simulink model "c2000_encode_decode_packet"  (R2021b)
settings: Solver=FixedStepDiscrete  StartTime=0.0  StopTime=Inf  RelTol=1e-3  EnableMultiTasking=on
undefined symbols (not defined in the file or in its folder): CR
libraries: embeddedblockslib x2, c280xlib x2, demo_controls x1
settings Model: ExtModeTrigDuration=8  Creator=The MathWorks, Inc.  LastModifiedBy=The MathWorks, Inc.
settings DataIOCC: ReturnWorkspaceOutputs=off
settings OptimizationCC: DefaultUnderspecifiedDataType=single  EnhancedBackFolding=on  PassReuseOutputArgsAs=Individual arguments  MaxStackSize=1024  OptimizeBlockOrder=speed  DifferentSizesBufferReuse=on  OptimizationCustomize=off  DenormalBehavior=FlushToZero  EfficientTunableParamExpr=on
settings DebuggingCC: ParameterPrecisionLossMsg=none  ParameterTunabilityLossMsg=error
settings HardwareCC: ProdBitPerChar=16  ProdBitPerInt=16  ProdBitPerPointer=32  ProdBitPerSizeT=32  ProdBitPerPtrDiffT=32  ProdLargestAtomicInteger=Integer  ProdLargestAtomicFloat=None  ProdWordSize=16  ProdLongLongMode=on  ProdHWDeviceType=Texas Instruments->C2000
settings ModelReferenceCC: ModelReferenceNumInstancesAllowed=Single
settings SFSimCC: MATLABDynamicMemAlloc=off
settings RTWCC: Description=Embedded Coder  SystemTargetFile=ert.tlc  HardwareBoard=TI Delfino F28379D LaunchPad  TemplateMakefile=ert_default_tmf  Toolchain=Texas Instruments Code Composer Studio (C2000)  BuildConfiguration=Faster Runs
settings CodeAppCC: ForceParamTrailComments=on  IgnoreCustomStorageClasses=off  OperatorAnnotations=on  SimulinkDataObjDesc=on  SFDataObjDesc=on  InsertBlockDesc=on
settings ERTTargetCC: CodeReplacementLibrary=TI C28x  ExtModeTransport=4  ExtModeStaticAlloc=on  ExtModeStaticAllocSize=10000  ExtModeMexFile=ext_xcp  ExtModeIntrfLevel=Level2 - Open

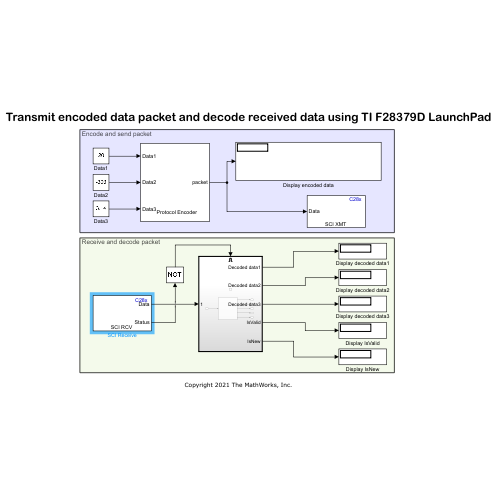
[thumbnail: Simulink's stored preview of the top-level diagram]
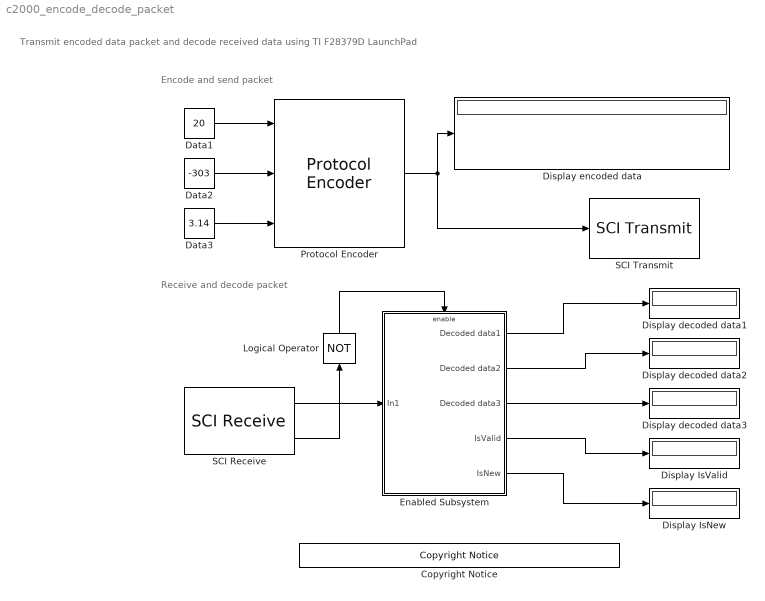
== system c2000_encode_decode_packet ==
  note: Receive and decode packet
  note: Transmit encoded data packet and decode received data using TI F28379D LaunchPad
  note: Encode and send packet
  Copyright Notice : demo_controls/Copyright Notice  year=2021  prod=tic6000
      settings: SourceProductBaseCode=ME
  Data1 : Constant  Value=20  OutDataTypeStr=uint8
  Data2 : Constant  Value=-303  OutDataTypeStr=int16
  Data3 : Constant  Value=3.14  OutDataTypeStr=single  LockScale=on
  Display IsNew : Display
  Display IsValid : Display
  Display decoded data1 : Display
  Display decoded data2 : Display
  Display decoded data3 : Display
  Display encoded data : Display
  Enabled Subsystem : Subsystem  TreatAsAtomicUnit=on
  Logical Operator : Logic  Operator=NOT  AllPortsSameDT=off  OutDataTypeStr=boolean
  Protocol Encoder : embeddedblockslib/Protocol Encoder  Header=36  FieldTable={ 'Data1', '1', 'uint8', 'Little endian'; 'Data2', '1', 'int16', 'Little endian'; 'Data3', '1', 'single', 'Little endian' }  IsChecksumRequired=on  ChecksumAlgorithm=XOR of bytes  ChecksumSize=[]  TerminatorOption=CR ('\r')  CustomTerminatorVal=[]
      settings: SourceProductBaseCode=ARDUINO,TIC2000
  SCI Receive : c280xlib/SCI Receive  sciModule=B  dataHead=''  dataTail=''  dataType=uint8  dataDim=10  initValue=0  errOption=Output the last received value  errValue=0  sampleTime=0.1  outputStatus=on  postInterrupt=off  numFifo=1
      settings: SourceProductBaseCode=TIC2000
  SCI Transmit : c280xlib/SCI Transmit  sciModule=B  dataHead=''  dataTail=''  postInterrupt=off  numFifo=1
  wires:
  Enabled Subsystem/3(Decoded data3) -> Display decoded data3/1
  Enabled Subsystem/1(Decoded data1) -> Display decoded data1/1
  Protocol Encoder/1 -> SCI Transmit/1, Display encoded data/1
  Enabled Subsystem/5(IsNew) -> Display IsNew/1
  Data3/1 -> Protocol Encoder/3
  Data1/1 -> Protocol Encoder/1
  Enabled Subsystem/4(IsValid) -> Display IsValid/1
  Enabled Subsystem/2(Decoded data2) -> Display decoded data2/1
  Data2/1 -> Protocol Encoder/2
  Logical Operator/1 -> Enabled Subsystem/Enable
  SCI Receive/1 -> Enabled Subsystem/1(In1)
  SCI Receive/2 -> Logical Operator/1

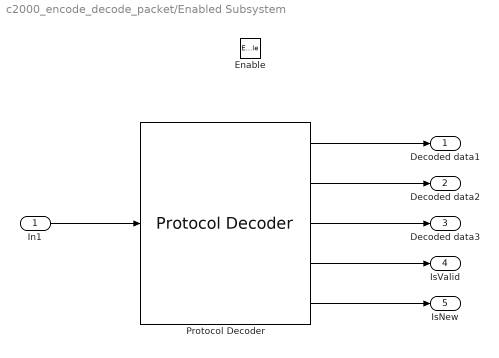
== system c2000_encode_decode_packet/Enabled Subsystem ==
  In1 : Inport
  Enable : EnablePort
  Protocol Decoder : embeddedblockslib/Protocol Decoder  IsParseCSV=off  Header=36  FieldTable={ 'Data1', '1', 'uint8', 'Little endian'; 'Data2', '1', 'int16', 'Little endian'; 'Data3', '1', 'single', 'Little endian' }  IsVariableSizeLastField=off  MaxVariableSizeFieldLength=[]  IsChecksumRequired=on  ChecksumAlgorithm=XOR of bytes  ChecksumSize=[]  TerminatorOption=CR ('\r')  CustomTerminatorVal=[]  IsInputLengthAvailable=off
      settings: SourceProductBaseCode=ARDUINO,TIC2000
  Decoded data1 : Outport
  Decoded data2 : Outport  Port=2
  Decoded data3 : Outport  Port=3
  IsValid : Outport  Port=4
  IsNew : Outport  Port=5
  wires:
  Protocol Decoder/3 -> Decoded data3/1
  In1/1 -> Protocol Decoder/1
  Protocol Decoder/2 -> Decoded data2/1
  Protocol Decoder/4 -> IsValid/1
  Protocol Decoder/1 -> Decoded data1/1
  Protocol Decoder/5 -> IsNew/1
